simulink model "sfbus_demo"  (R2017b)
settings: Solver=FixedStepDiscrete  StartTime=0.0  StopTime=10  RelTol=1e-3  EnableMultiTasking=on
PreLoadFcn:
  | load bus_objects;
settings Model: ExtModeAutoUpdateStatusClock=off  Creator=The MathWorks, Inc.  LastModifiedBy=The MathWorks, Inc.
settings DataIOCC: LimitDataPoints=on  SaveFormat=Structure  SignalLogging=off  SaveTime=off
settings OptimizationCC: DefaultParameterBehavior=Inlined  InlineInvariantSignals=on  ExpressionDepthLimit=2147483647  InitFltsAndDblsToZero=on  EfficientMapNaN2IntZero=off  LifeSpan=inf
settings DebuggingCC: SaveWithParameterizedLinksMsg=none  UnderspecifiedInitializationDetection=Classic  MergeDetectMultiDrivingBlocksExec=none  MultiTaskDSMMsg=warning  MultiTaskCondExecSysMsg=none  FcnCallInpInsideContextMsg=warning  StateNameClashWarn=warning  SFUnexpectedBacktrackingDiag=warning  SFNoUnconditionalDefaultTransitionDiag=warning  SFExecutionAtInitializationDiag=none
settings HardwareCC: ProdBitPerPointer=32  ProdBitPerSizeT=32  ProdBitPerPtrDiffT=32  ProdLargestAtomicFloat=None  ProdIntDivRoundTo=Undefined  ProdEndianess=Unspecified  ProdWordSize=32  ProdHWDeviceType=32-bit Generic
settings ModelReferenceCC: PropagateSignalLabelsOutOfModel=off
settings SFSimCC: SimCustomHeaderCode="#include \"counterbus.h\""  SimUserSources=counterbus.c  SimParseCustomCode=off
settings RTWCC: Description=Generic Real-Time Target  CustomSource=counterbus.c
settings CodeAppCC: StateflowObjectComments=on
settings GRTTargetCC: TargetFcnLib=ansi_tfl_tmw.mat  TargetLangStandard=C89/C90 (ANSI)  GeneratePreprocessorConditionals=Disable all  CombineOutputUpdateFcns=off  GRTInterface=on
settings ConfigComp: CovMetricSettings=dw  CovHtmlReporting=on  CovSaveCumulativeToWorkspaceVar=on  CovSaveSingleToWorkspaceVar=on  CovExternalEMLEnable=off  CovSFcnEnable=off

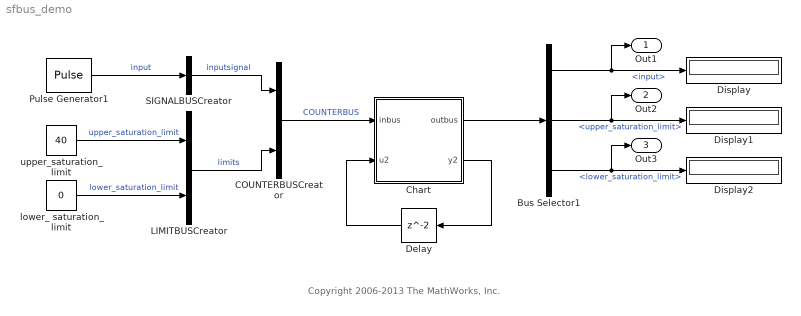
== system sfbus_demo ==
  note: Copyright 2006-2013 The MathWorks, Inc.
  Bus Selector1 : BusSelector  OutputSignals=inputsignal.input,limits.upper_saturation_limit,limits.lower_saturation_limit
  COUNTERBUSCreator : BusCreator  Inputs=2  OutDataTypeStr=Bus: COUNTERBUS  NonVirtualBus=on
  Chart : Stateflow chart  TreatAsAtomicUnit=on
  Delay : Delay
  Display : Display
      settings: Format=short_e
  Display1 : Display
      settings: Format=short_e
  Display2 : Display
      settings: Format=short_e
  LIMITBUSCreator : BusCreator  Inputs=2  OutDataTypeStr=Bus: LIMITBUS  NonVirtualBus=on
  Pulse Generator1 : DiscretePulseGenerator  Amplitude=int32(1)  SampleTime=0.1
  SIGNALBUSCreator : BusCreator  Inputs=1  OutDataTypeStr=Bus: SIGNALBUS  NonVirtualBus=on
  lower_ saturation_ limit : Constant  Value=0  OutDataTypeStr=int32
  upper_saturation_limit : Constant  Value=40  OutDataTypeStr=int32
  Out1 : Outport
  Out2 : Outport  Port=2
  Out3 : Outport  Port=3
  wires:
  upper_saturation_limit/1 -> LIMITBUSCreator/1  "upper_saturation_limit"
  lower_ saturation_ limit/1 -> LIMITBUSCreator/2  "lower_saturation_limit"
  Pulse Generator1/1 -> SIGNALBUSCreator/1  "input"
  LIMITBUSCreator/1 -> COUNTERBUSCreator/2  "limits"
  SIGNALBUSCreator/1 -> COUNTERBUSCreator/1  "inputsignal"
  COUNTERBUSCreator/1 -> Chart/1(inbus)  "COUNTERBUS"
  Chart/2(y2) -> Delay/1
  Delay/1 -> Chart/2(u2)
  Chart/1(outbus) -> Bus Selector1/1
  Bus Selector1/1 -> Display/1, Out1/1  "<input>"
  Bus Selector1/2 -> Display1/1, Out2/1  "<upper_saturation_limit>"
  Bus Selector1/3 -> Display2/1, Out3/1  "<lower_saturation_limit>"

== stateflow chart sfbus_demo/Chart ==
  state y = get_input_signal(u) [function]
    (default) -> (junction 5) : { y = u.inputsignal; }
  (default) -> (junction 4) : {
      | counterbus_struct = inbus;
      | counterbus_struct.inputsignal = get_input_signal(inbus);
      |
      | counterbusFcn(&counterbus_struct, u2, &outbus, &y2);
      | }
  data: u function_input Bus: COUNTERBUS size=1 =0; y function_output Bus: SIGNALBUS size=1 =0; inbus input Bus: COUNTERBUS size=1; outbus output Bus: COUNTERBUS size=1 =0; u2 input int32; y2 output int32; counterbus_struct local type(inbus)
